simulink model "week3_P3"  (R2020b)
settings: Solver=VariableStepAuto  StartTime=0.0  StopTime=10.0  RelTol=1e-3
model workspace (MAT data in the model file):
  I = 5
  Kf = 1
  PBmax = 1500
  Rr = 1.25
  TB = 0.01
  ctrl = 1
  g = 32.18
  m = 50
  mu = [0 0.4 0.8 0.97 1 0.98 0.96 0.94 0.92 0.9 0.88 0.855 0.83 0.81 0.79 0.77 0.75 0.73 0.72 0.71 0.7]
  slip = [0 0.05 0.1 0.15 0.2 0.25 0.3 0.35 0.4 0.45 0.5 0.55 0.6 0.65 0.7 0.75 0.8 0.85 0.9 0.95 1]
  v0 = 88
settings Model: DataDictionary=Var1.sldd  OrderedModelArguments=off  Creator=ADMIN  LastModifiedBy=ADMIN

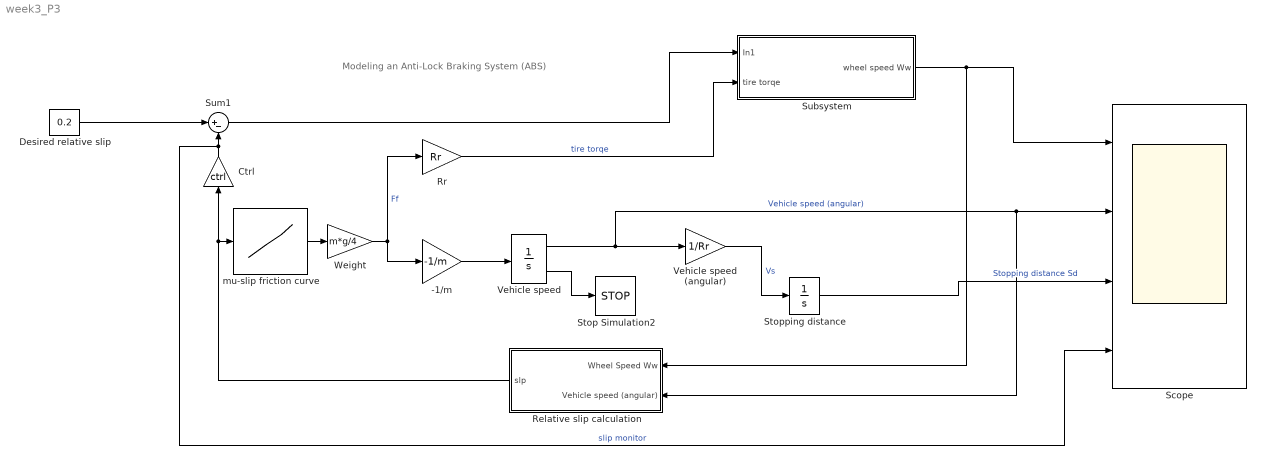
== system week3_P3 ==
  note: Modeling an Anti-Lock Braking System (ABS)
  -1/m : Gain  Gain=-1/m  SaturateOnIntegerOverflow=on  OutDataTypeStr=Inherit: Same as input  ParamDataTypeStr=Inherit: Same as input
  Ctrl : Gain  Gain=ctrl  SaturateOnIntegerOverflow=on  OutDataTypeStr=Inherit: Same as input  ParamDataTypeStr=Inherit: Same as input
  Desired relative slip : Constant  Value=0.2
  Relative slip calculation : Subsystem
  Rr : Gain  Gain=Rr  SaturateOnIntegerOverflow=on  OutDataTypeStr=Inherit: Same as input  ParamDataTypeStr=Inherit: Same as input
  Scope : Scope  NumInputPorts=4
  Stop Simulation2 : Stop
  Stopping distance : Integrator  UpperSaturationLimit=1000  LowerSaturationLimit=0
  Subsystem : Subsystem
  Sum1 : Sum  Inputs=|+-  InputSameDT=on  SaturateOnIntegerOverflow=on  OutDataTypeStr=Inherit: Same as first input
  Vehicle speed : Integrator  InitialCondition=v0  LimitOutput=on  UpperSaturationLimit=1000  LowerSaturationLimit=0  ShowSaturationPort=on
  Vehicle speed (angular) : Gain  Gain=1/Rr  SaturateOnIntegerOverflow=on  OutDataTypeStr=Inherit: Same as input  ParamDataTypeStr=Inherit: Same as input
  Weight : Gain  Gain=m*g/4  SaturateOnIntegerOverflow=on  OutDataTypeStr=Inherit: Same as input  ParamDataTypeStr=Inherit: Same as input
  mu-slip friction curve : Lookup_n-D  NumberOfTableDimensions=1  BreakpointsForDimension1=slip  Table=mu  SaturateOnIntegerOverflow=on  InputSameDT=on
  wires:
  -1/m/1 -> Vehicle speed/1
  Desired relative slip/1 -> Sum1/1
  Vehicle speed (angular)/1 -> Stopping distance/1  "Vs"
  Ctrl/1 -> Scope/4, Sum1/2  "slip monitor"
  Stopping distance/1 -> Scope/3  "Stopping distance Sd"
  Relative slip calculation/1(slp) -> Ctrl/1, mu-slip friction curve/1
  Rr/1 -> Subsystem/2(tire torqe)  "tire torqe"
  mu-slip friction curve/1 -> Weight/1
  Subsystem/1(wheel speed Ww) -> Relative slip calculation/1(Wheel Speed Ww), Scope/1
  Sum1/1 -> Subsystem/1(In1)
  Vehicle speed/2 -> Stop Simulation2/1
  Weight/1 -> Rr/1, -1/m/1  "Ff"
  Vehicle speed/1 -> Relative slip calculation/2(Vehicle speed (angular)), Scope/2, Vehicle speed (angular)/1  "Vehicle speed (angular)"

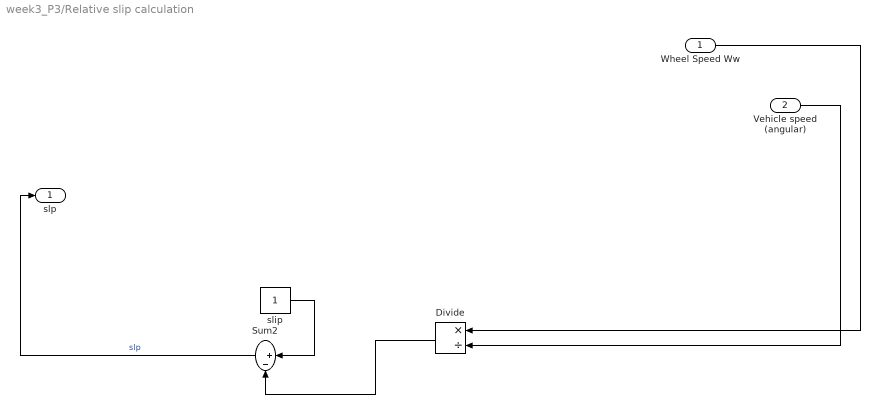
== system week3_P3/Relative slip calculation ==
  Wheel Speed Ww : Inport
  Vehicle speed (angular) : Inport  Port=2
  Divide : Product  Inputs=*/
  Sum2 : Sum  Inputs=|+-  InputSameDT=on  SaturateOnIntegerOverflow=on  OutDataTypeStr=Inherit: Same as first input
  slip : Constant
  slp : Outport
  wires:
  Divide/1 -> Sum2/2
  slip/1 -> Sum2/1
  Wheel Speed Ww/1 -> Divide/1
  Vehicle speed (angular)/1 -> Divide/2
  Sum2/1 -> slp/1  "slp"

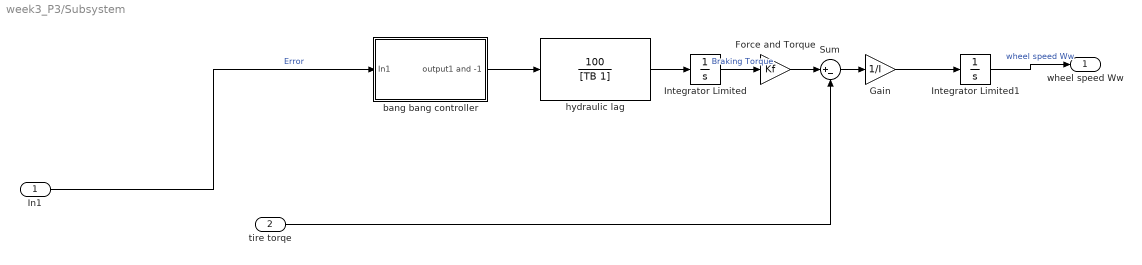
== system week3_P3/Subsystem ==
  In1 : Inport
  tire torqe : Inport  Port=2
  Force and Torque : Gain  Gain=Kf
  Gain : Gain  Gain=1/I
  Integrator Limited : Integrator  LimitOutput=on  UpperSaturationLimit=PBmax  LowerSaturationLimit=0
  Integrator Limited1 : Integrator  InitialCondition=v0/Rr  LimitOutput=on  UpperSaturationLimit=1000  LowerSaturationLimit=0
  Sum : Sum  Inputs=|+-
  bang bang controller : Subsystem
  hydraulic lag : TransferFcn  Numerator=[100]  Denominator=[TB 1]
  wheel speed Ww : Outport
  wires:
  Integrator Limited1/1 -> wheel speed Ww/1  "wheel speed Ww"
  hydraulic lag/1 -> Integrator Limited/1
  tire torqe/1 -> Sum/2
  Gain/1 -> Integrator Limited1/1
  bang bang controller/1(output1 and -1) -> hydraulic lag/1
  Sum/1 -> Gain/1
  In1/1 -> bang bang controller/1(In1)  "Error"
  Force and Torque/1 -> Sum/1
  Integrator Limited/1 -> Force and Torque/1  "Braking Torque"

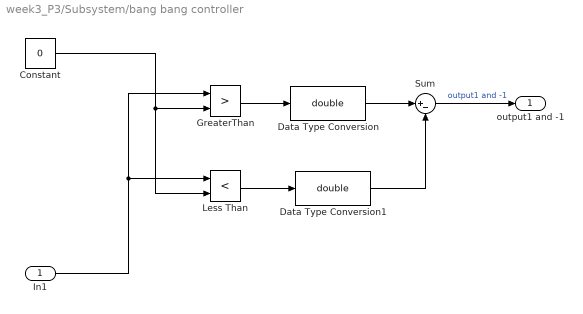
== system week3_P3/Subsystem/bang bang controller ==
  In1 : Inport
  Constant : Constant  Value=0
  Data Type Conversion : DataTypeConversion  OutDataTypeStr=double  RndMeth=Zero
  Data Type Conversion1 : DataTypeConversion  OutDataTypeStr=double  RndMeth=Zero
  GreaterThan : RelationalOperator  Operator=>  OutDataTypeStr=boolean  RndMeth=Simplest
  Less Than : RelationalOperator  Operator=<  OutDataTypeStr=boolean  RndMeth=Simplest
  Sum : Sum  Inputs=|+-
  output1 and -1 : Outport
  wires:
  GreaterThan/1 -> Data Type Conversion/1
  Constant/1 -> Less Than/2, GreaterThan/2
  Sum/1 -> output1 and -1/1  "output1 and -1"
  In1/1 -> Less Than/1, GreaterThan/1
  Data Type Conversion/1 -> Sum/1
  Less Than/1 -> Data Type Conversion1/1
  Data Type Conversion1/1 -> Sum/2
